simulink library "ESTS_VVSO_WHL_LgtLoadTransf"  (R2024b)
settings: Solver=VariableStepAuto  StartTime=0.0  StopTime=10.0  RelTol=1e-3
settings Model: Creator=blatak  LastModifiedBy=blatak
settings ModelReferenceCC: EnableRefExpFcnMdlSchedulingChecks=on
settings RTWCC: GPUComputeCapability=3.5

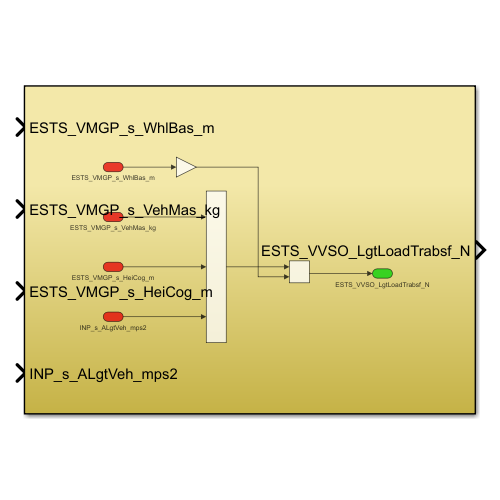
[thumbnail: Simulink's stored preview of the top-level diagram]
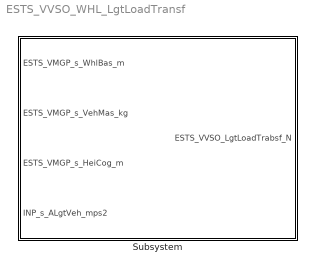
== system ESTS_VVSO_WHL_LgtLoadTransf ==
  Subsystem : Subsystem

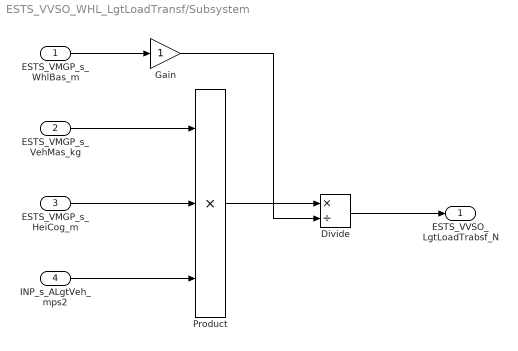
== system ESTS_VVSO_WHL_LgtLoadTransf/Subsystem ==
  ESTS_VMGP_s_WhlBas_m : Inport
  ESTS_VMGP_s_VehMas_kg : Inport  Port=2
  ESTS_VMGP_s_HeiCog_m : Inport  Port=3
  INP_s_ALgtVeh_mps2 : Inport  Port=4
  Divide : Product  Inputs=*/  RndMeth=Zero  SaturateOnIntegerOverflow=on
  Gain : Gain
  Product : Product  Inputs=3
  ESTS_VVSO_LgtLoadTrabsf_N : Outport
  wires:
  ESTS_VMGP_s_VehMas_kg/1 -> Product/1
  INP_s_ALgtVeh_mps2/1 -> Product/3
  ESTS_VMGP_s_HeiCog_m/1 -> Product/2
  Product/1 -> Divide/1
  ESTS_VMGP_s_WhlBas_m/1 -> Gain/1
  Divide/1 -> ESTS_VVSO_LgtLoadTrabsf_N/1
  Gain/1 -> Divide/2
